simulink model "Octocopter2D_04States"  (R2020b)
settings: Solver=VariableStepAuto  StartTime=0.0  StopTime=10  MaxStep=1e-3  RelTol=1e-3
undefined symbols (not defined in the file): Uav
libraries: simulink_extras x4
settings Model: Creator=jeremie  LastModifiedBy=jeremie
settings DebuggingCC: ArithmeticOperatorsInVariantConditions=warning
settings SFSimCC: SimUseLocalCustomCode=off  CustomCodeUndefinedFunction=UseInterfaceOnly
settings RTWCC: RTWUseLocalCustomCode=off

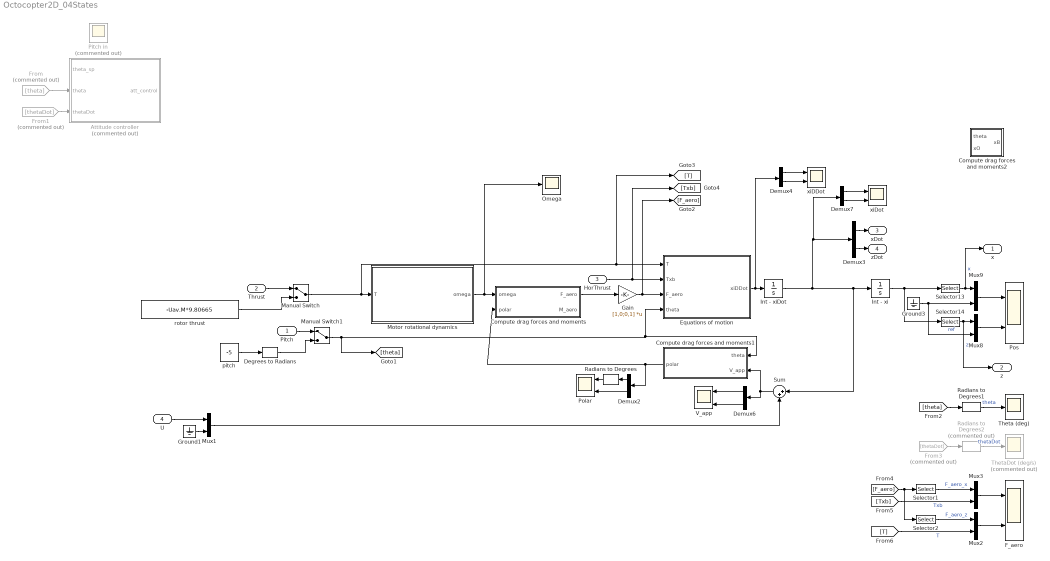
== system Octocopter2D_04States ==
  Pitch : Inport
  Thrust : Inport  Port=2
  HorThrust : Inport  Port=3
  U : Inport  Port=4
  Attitude controller : Subsystem  Commented=on
  Compute drag forces and moments : MATLAB Function  TreatAsAtomicUnit=on
  Compute drag forces and moments1 : MATLAB Function  TreatAsAtomicUnit=on
  Compute drag forces and moments2 : MATLAB Function  TreatAsAtomicUnit=on
  Degrees to Radians : simulink_extras/Transformations/Degrees to Radians
  Demux{2..4,6..7} (5 alike) : Demux  Outputs=2
  Equations of motion : MATLAB Function  TreatAsAtomicUnit=on
  F_aero : Scope  NumInputPorts=2
  From : From  Commented=on  GotoTag=theta
  From1 : From  Commented=on  GotoTag=thetaDot
  From3 : From  Commented=on  GotoTag=thetaDot
  Gain : Gain  Gain=[1,0;0,1]  Multiplication=Matrix(K*u)
  Ground1 : Ground
  Ground3 : Ground
  Int - xi : Integrator  ContinuousStateAttributes={'x','z'}
  Int - xiDot : Integrator  ContinuousStateAttributes={'xDot','zDot'}
  Manual Switch : ManualSwitch
  Manual Switch1 : ManualSwitch
  Motor rotational dynamics : MATLAB Function  TreatAsAtomicUnit=on
  Mux{1..3,8..9} (5 alike) : Mux  Inputs=2
  Omega : Scope
  Pitch in : Scope  Commented=on
  Polar : Scope  NumInputPorts=2
  Pos : Scope  NumInputPorts=2
  Radians to Degrees : simulink_extras/Transformations/Radians to Degrees
  Radians to Degrees1 : simulink_extras/Transformations/Radians to Degrees
  Radians to Degrees2 : simulink_extras/Transformations/Radians to Degrees  Commented=on
  Selector1 : Selector  InputPortWidth=2  IndexOptions=Index vector (dialog)  Indices=1  OutputSizes=1
  Selector13 : Selector  InputPortWidth=2  IndexOptions=Index vector (dialog)  Indices=1  OutputSizes=1
  Selector14 : Selector  InputPortWidth=2  IndexOptions=Index vector (dialog)  Indices=2  OutputSizes=1
  Selector2 : Selector  InputPortWidth=2  IndexOptions=Index vector (dialog)  Indices=2  OutputSizes=1
  Sum : Sum  Inputs=|++
  Theta (deg) : Scope
  ThetaDot (deg/s) : Scope  Commented=on
  V_app : Scope  NumInputPorts=2
  pitch : Constant  Value=-5
  rotor thrust : Constant  Value=-Uav.M*9.80665
  xiDDot : Scope  NumInputPorts=2
  xiDot : Scope  NumInputPorts=2
  x : Outport  VectorParamsAs1DForOutWhenUnconnected=off
  z : Outport  Port=2  VectorParamsAs1DForOutWhenUnconnected=off
  xDot : Outport  Port=3  VectorParamsAs1DForOutWhenUnconnected=off
  zDot : Outport  Port=4  VectorParamsAs1DForOutWhenUnconnected=off
  wires:
  Motor rotational dynamics/1(omega) -> Compute drag forces and moments/1(omega), Omega/1
  Compute drag forces and moments/1(F_aero) -> Gain/1
  Manual Switch/1 -> Equations of motion/1(T), [T], Motor rotational dynamics/1(T)
  Equations of motion/1(xiDDot) -> Demux4/1, Int - xiDot/1
  Mux1/1 -> Sum/2
  Sum/1 -> Compute drag forces and moments1/2(V_app), Demux6/1
  Compute drag forces and moments1/1(polar) -> Demux2/1, Compute drag forces and moments/2(polar)
  Ground3/1 -> Mux8/2, Mux9/2  "ref"
  Selector14/1 -> z/1, Mux8/1  "z"
  Selector13/1 -> x/1, Mux9/1  "x"
  Mux8/1 -> Pos/2
  Mux9/1 -> Pos/1
  Int - xi/1 -> Selector14/1, Selector13/1
  Demux2/2 -> Polar/2
  Demux2/1 -> Radians to Degrees/1
  Radians to Degrees/1 -> Polar/1
  Radians to Degrees1/1 -> Theta (deg)/1  "theta"
  From/1 -> Attitude controller/2(theta)
  From1/1 -> Attitude controller/3(thetaDot)
  HorThrust/1 -> [Txb], Equations of motion/2(Txb)
  [theta] -> Radians to Degrees1/1
  Demux3/1 -> xDot/1
  Demux3/2 -> zDot/1
  Demux4/1 -> xiDDot/1
  Demux4/2 -> xiDDot/2
  From3/1 -> Radians to Degrees2/1
  Radians to Degrees2/1 -> ThetaDot (deg/s)/1  "thetaDot"
  U/1 -> Mux1/1
  Ground1/1 -> Mux1/2
  Mux3/1 -> F_aero/1
  Selector1/1 -> Mux3/1  "F_aero_x"
  [F_aero] -> Selector2/1, Selector1/1
  Thrust/1 -> Manual Switch/1
  rotor thrust/1 -> Manual Switch/2
  Pitch/1 -> Manual Switch1/1
  pitch/1 -> Degrees to Radians/1
  Demux6/1 -> V_app/1
  Demux6/2 -> V_app/2
  Demux7/2 -> xiDot/2
  Demux7/1 -> xiDot/1
  Int - xiDot/1 -> Demux7/1, Demux3/1, Sum/1, Int - xi/1
  Gain/1 -> [F_aero], Equations of motion/3(F_aero)
  Manual Switch1/1 -> [theta], Equations of motion/4(theta), Compute drag forces and moments1/1(theta)
  [Txb] -> Mux3/2  "Txb"
  Mux2/1 -> F_aero/2
  Selector2/1 -> Mux2/1  "F_aero_z"
  [T] -> Mux2/2  "T"
  Degrees to Radians/1 -> Manual Switch1/2

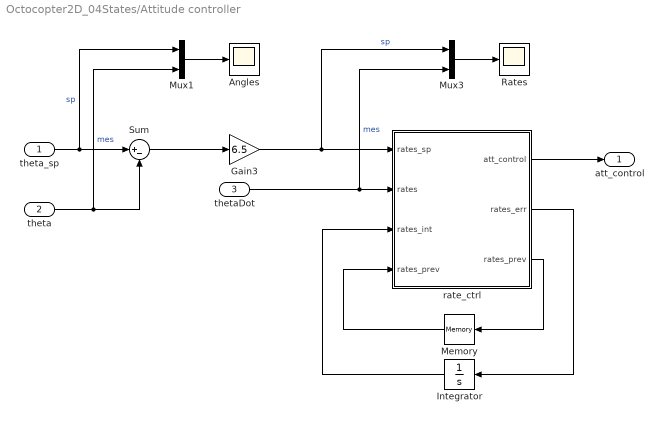
== system Octocopter2D_04States/Attitude controller ==
  theta_sp : Inport
  theta : Inport  Port=2
  thetaDot : Inport  Port=3
  Angles : Scope
  Gain3 : Gain  Gain=6.5
  Integrator : Integrator
  Memory : Memory
  Mux1 : Mux  Inputs=2
  Mux3 : Mux  Inputs=2
  Rates : Scope
  Sum : Sum  Inputs=|+-
  rate_ctrl : MATLAB Function  TreatAsAtomicUnit=on  SystemSampleTime=0.002
  att_control : Outport  VectorParamsAs1DForOutWhenUnconnected=off
  wires:
  rate_ctrl/2(rates_err) -> Integrator/1
  rate_ctrl/3(rates_prev) -> Memory/1
  Integrator/1 -> rate_ctrl/3(rates_int)
  rate_ctrl/1(att_control) -> att_control/1
  Memory/1 -> rate_ctrl/4("rates_prev ")
  Mux3/1 -> Rates/1
  thetaDot/1 -> rate_ctrl/2(rates), Mux3/2  "mes"
  Gain3/1 -> rate_ctrl/1(rates_sp), Mux3/1  "sp"
  Sum/1 -> Gain3/1
  theta_sp/1 -> Mux1/1, Sum/1  "sp"
  theta/1 -> Mux1/2, Sum/2  "mes"
  Mux1/1 -> Angles/1

== matlab function Octocopter2D_04States/Attitude controller/rate_ctrl ==
  data: rates_sp input size=1; rates input size=1; att_control output size=1; rates_err output; rates_prev output; rates_int input size=1; rates_prev input size=1
function [ att_control, rates_err, rates_prev ] = rate_ctrl(rates_sp, rates, rates_int, rates_prev)
rates_p = 0.15;
rates_i = 0.05;
rates_d = 0.003;
rate_ff = 0;

dt = 0.002;

% Angular rates error
rates_err = - rates_sp + rates;

% % Perform the integration using a first order method and do not propaate the result if out of range or invalid
% rates_int = rates_int +  rates_err * dt;

att_control = rates_p .* rates_err + rates_i .* rates_int + rates_d .* (rates_prev - rates) ./ dt + rate_ff .* rates_sp;

rates_prev = rates;

end

== matlab function Octocopter2D_04States/Compute drag forces and moments2 ==
  data: theta input; xO input; xB output
function xB   = O2B( theta, xO )
%#codegen

xB = [ cos(theta), -sin(theta); sin(theta), cos(theta) ] * xO;

== matlab function Octocopter2D_04States/Compute drag forces and moments ==
  data: omega input; polar input size=2; F_aero output; M_aero output; Uav parameter
function [F_aero, M_aero] = computeAero( omega, polar, Uav )
%#codegen

% Name variables
alpha    = -polar(1); % equations assume alpha measured the other way
U        = polar(2);
omegaBar = mean(omega);
rho      = Uav.RHO_AIR;
D_UAV    = Uav.D_UAV;
A_UAV    = Uav.A_UAV;
D_PROP   = Uav.D_PROP;
A_PROP   = Uav.A_PROP;
n        = Uav.N_ROTORS;

% Force coefficients
Cxb1 = -0.241*cos(alpha) + 0.036*cos(3*alpha) + 0.016*cos(7*alpha);
Cxb2 = -0.053*cos(alpha) - 0.008*cos(3*alpha);
Czb1 = -0.724*sin(alpha) + 0.080;
Czb2 = -0.222*sin(alpha) + 0.065;

% Moment coefficients
lambda = omegaBar*D_PROP / ( 2*U );
A1  =  0.116 * ( 1 - exp(-0.126*lambda) );
A2  = -0.041 * ( 1 - exp(-0.308*lambda) );
CM1 =  0.009*cos(alpha) + 0.003*cos(3*alpha) - 0.014*sin(2*alpha);
CM2 =  A1*cos(alpha) + A2*sin(2*alpha);

% Forces and moments
Fxb = 0.5*rho*U^2*Cxb1*A_UAV      + 0.5*rho*U*omegaBar*Cxb2*D_PROP*A_PROP*(n/4);
Fzb = 0.5*rho*U^2*Czb1*A_UAV      + 0.5*rho*U*omegaBar*Czb2*D_PROP*A_PROP*(n/4);
M   = 0.5*rho*U^2*CM1*A_UAV*D_UAV + 0.5*rho*U*omegaBar*CM2*D_PROP^2*A_PROP*(n/4);

% Output forces - NED
F_aero = [ Fxb; -Fzb ];
M_aero = M;

== matlab function Octocopter2D_04States/Motor rotational dynamics ==
  data: T input; omega output; Uav parameter
function omega = motorRotDynamics( T, Uav )
%#codegen

omega = sqrt( sqrt(T^2)/(cos(Uav.ZETA)*Uav.C_T) );

== matlab function Octocopter2D_04States/Equations of motion ==
  data: T input; Txb input; xiDDot output; F_aero input size=2; theta input; Uav parameter
function xiDDot   = Octo2DModel( T, Txb, F_aero, theta, Uav )
%#codegen

% Name variables
m_UAV = Uav.M;
Fxb = F_aero(1);
Fzb = F_aero(2);
g = 9.80665;

% Forces and pitching moment in world frame
xDDot = ( (T + Fzb)*sin(theta) + (Txb + Fxb)*cos(theta) ) / m_UAV;
zDDot = ( (T + Fzb)*cos(theta) + (Txb + Fxb)*sin(theta) + m_UAV*g ) / m_UAV;

xiDDot = [xDDot; zDDot];

end

== matlab function Octocopter2D_04States/Compute drag forces and moments1 ==
  data: theta input; V_app input; polar output
function polar   = computeSph( theta, V_app )
%#codegen

V_appBody = [ cos(theta), -sin(theta); sin(theta), cos(theta) ] * V_app; % CHECK

% alpha = theta since wind is horizontal
polar = [atan2(V_appBody(2), V_appBody(1)); norm(V_appBody)];
